simulink model "PAM_Timing"  (R2016a)
settings: Solver=VariableStepAuto  StartTime=0.0  StopTime=(12+256+8+602)*8  RelTol=1e-3
undefined symbols (not defined in the file or in its folder): rcosine
settings Model: Creator=coltmt  LastModifiedBy=coltmt

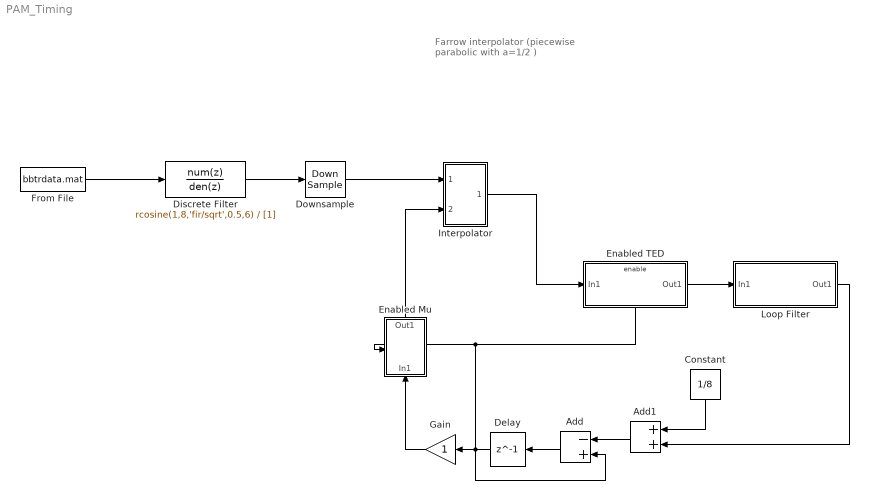
== system PAM_Timing ==
  note: Farrow interpolator (piecewise parabolic with a=1/2 )
  Add : Sum  Inputs=-+
  Add1 : Sum
  Constant : Constant  Value=1/8
  Delay : Delay  DelayLength=1
  Discrete Filter : DiscreteFilter  Numerator=rcosine(1,8,'fir/sqrt',0.5,6)  Denominator=[1]
  Downsample : DownSample  N=8/2
  Enabled Mu : Subsystem  TreatAsAtomicUnit=on
  Enabled TED : Subsystem  TreatAsAtomicUnit=on
  From File : FromFile  FileName=bbtrdata.mat  SampleTime=1
  Gain : Gain
  "Interpolator " : Subsystem
  "Loop Filter " : Subsystem
  wires:
  From File/1 -> Discrete Filter/1
  Discrete Filter/1 -> Downsample/1
  Downsample/1 -> "Interpolator "/1(In1)
  Add/1 -> Delay/1
  Delay/1 -> Enabled TED/Enable, Enabled Mu/Enable, Gain/1, Add/2
  Add1/1 -> Add/1
  Constant/1 -> Add1/1
  Enabled Mu/1(Out1) -> "Interpolator "/2(In2)
  Gain/1 -> Enabled Mu/1(In1)
  "Interpolator "/1(Out1) -> Enabled TED/1(In1)
  Enabled TED/1(Out1) -> "Loop Filter "/1(In1)
  "Loop Filter "/1(Out1) -> Add1/2

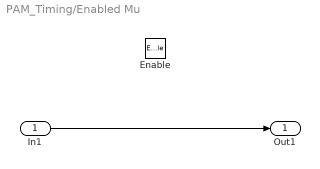
== system PAM_Timing/Enabled Mu ==
  In1 : Inport
  Enable : EnablePort
  Out1 : Outport
  wires:
  In1/1 -> Out1/1

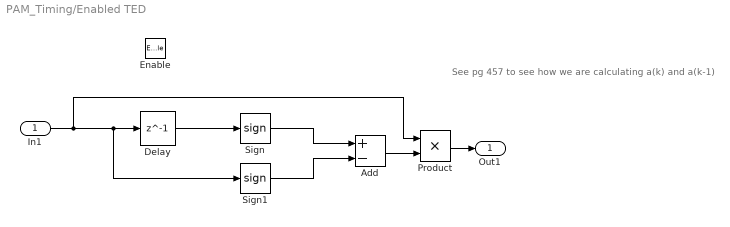
== system PAM_Timing/Enabled TED ==
  note: See pg 457 to see how we are calculating a(k) and a(k-1)
  In1 : Inport
  Enable : EnablePort  StatesWhenEnabling=reset
  Add : Sum  Inputs=+-
  Delay : Delay  DelayLength=1
  Product : Product
  Sign : Signum
  Sign1 : Signum
  Out1 : Outport
  wires:
  Add/1 -> Product/2
  In1/1 -> Sign1/1, Delay/1, Product/1
  Delay/1 -> Sign/1
  Sign/1 -> Add/1
  Sign1/1 -> Add/2
  Product/1 -> Out1/1

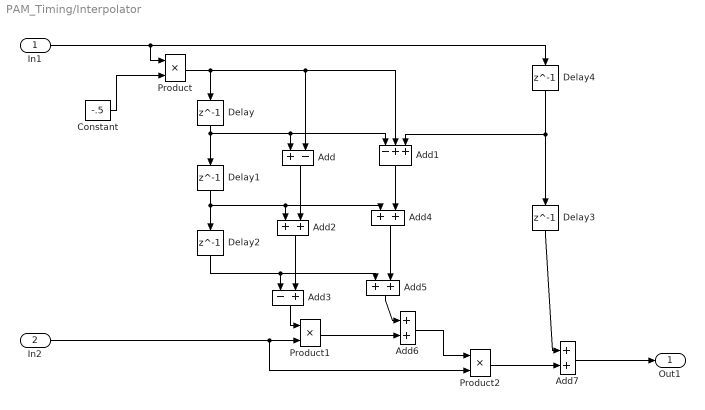
== system PAM_Timing/Interpolator  ==
  In1 : Inport
  In2 : Inport  Port=2
  Add : Sum  Inputs=+-
  Add1 : Sum  Inputs=-++
  Add{2,4..7} (5 alike) : Sum
  Add3 : Sum  Inputs=-+
  Constant : Constant  Value=-.5
  Delay{,1..4} (5 alike) : Delay  DelayLength=1  InputProcessing=Columns as channels (frame based)
  Product : Product
  Product1 : Product
  Product2 : Product
  Out1 : Outport
  wires:
  In1/1 -> Delay4/1, Product/1
  Constant/1 -> Product/2
  Add3/1 -> Product1/1
  Delay/1 -> Delay1/1, Add1/1, Add/1
  Delay2/1 -> Add5/1, Add3/1
  Add6/1 -> Product2/1
  Product/1 -> Add1/2, Add/2, Delay/1
  Delay4/1 -> Add1/3, Delay3/1
  Add5/1 -> Add6/1
  Add7/1 -> Out1/1
  Product2/1 -> Add7/2
  Add2/1 -> Add3/2
  Add1/1 -> Add4/2
  Add/1 -> Add2/2
  Product1/1 -> Add6/2
  Delay3/1 -> Add7/1
  Add4/1 -> Add5/2
  In2/1 -> Product2/2, Product1/2
  Delay1/1 -> Add4/1, Add2/1, Delay2/1

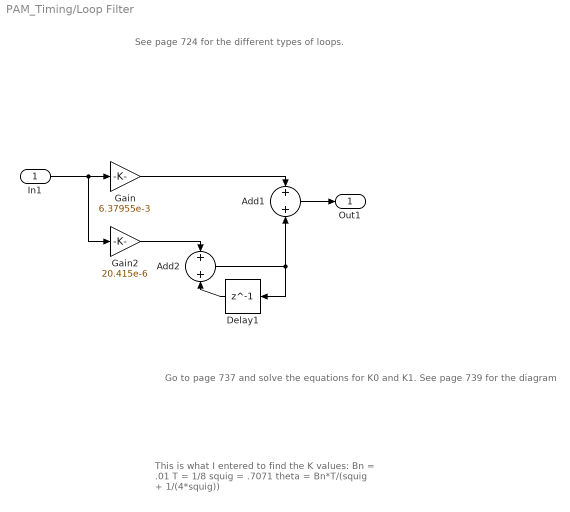
== system PAM_Timing/Loop Filter  ==
  note: This is what I entered to find the K values:
      | Bn = .01
      | T = 1/8
      | squig = .7071
      | theta = Bn*T/(squig + 1/(4*squig))
  note: See page 724 for the different types of loops.
  note: Go to page 737 and solve the equations for K0 and K1. See page 739 for the diagram
  In1 : Inport
  Add1 : Sum
  Add2 : Sum
  Delay1 : Delay  DelayLength=1
  Gain : Gain  Gain=6.37955e-3
  Gain2 : Gain  Gain=20.415e-6
  Out1 : Outport
  wires:
  Gain/1 -> Add1/1
  Delay1/1 -> Add2/2
  Add2/1 -> Add1/2, Delay1/1
  Gain2/1 -> Add2/1
  In1/1 -> Gain2/1, Gain/1
  Add1/1 -> Out1/1
